simulink model "VCU_CS75_9_30"  (R2014a)
settings: Solver=FixedStepDiscrete  StartTime=0.0  StopTime=25  FixedStep=0.0005  RelTol=1e-3
undefined symbols (not defined in the file or in its folder): APAStatus_2D4, ecucoder_acal, I_SW01_L, LDW, ST_comd, TX2D4
libraries: simulink x881, ec5744lib x37
(part 4 of 30)

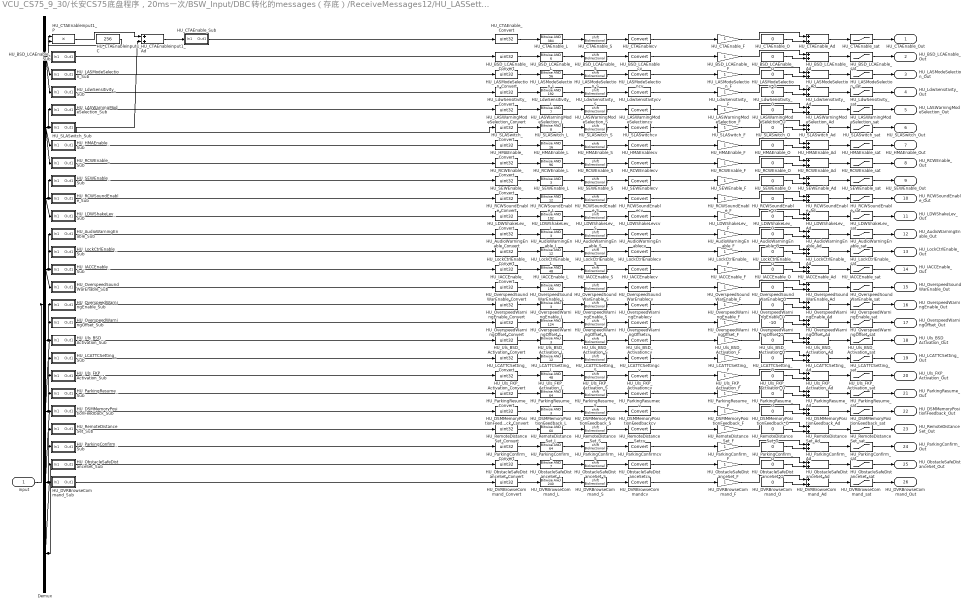
== system VCU_CS75_9_30/长安CS75底盘程序，20ms一次/BSW_Input/DBC转化的messages（存底）/ReceiveMessages12/HU_LASSetting_0x541 ==
  input : Inport
  Demux : Demux  Outputs=8
  HU_AudioWarningEnable_Ad : Sum
  HU_AudioWarningEnable_Convert : DataTypeConversion  OutDataTypeStr=uint32
  HU_AudioWarningEnable_F : Gain
  HU_AudioWarningEnable_L : simulink/Logic and Bit Operations/Bitwise Operator  logicop=AND  UseBitMask=on  BitMask=3  BitMaskRealWorld=Stored Integer
  HU_AudioWarningEnable_O : Constant  Value=0  OutDataTypeStr=single
  HU_AudioWarningEnable_S : ArithShift
  HU_AudioWarningEnable_Sub : Subsystem
  HU_AudioWarningEnable_sat : Saturate  UpperLimit=3  LowerLimit=0
  HU_AudioWarningEnablecv : DataTypeConversion
  HU_BSD_LCAEnable_Ad : Sum
  HU_BSD_LCAEnable_Convert : DataTypeConversion  OutDataTypeStr=uint32
  HU_BSD_LCAEnable_F : Gain
  HU_BSD_LCAEnable_L : simulink/Logic and Bit Operations/Bitwise Operator  logicop=AND  UseBitMask=on  BitMask=6  BitMaskRealWorld=Stored Integer
  HU_BSD_LCAEnable_O : Constant  Value=0  OutDataTypeStr=single
  HU_BSD_LCAEnable_S : ArithShift  BitShiftNumber=1
  HU_BSD_LCAEnable_Sub : Subsystem
  HU_BSD_LCAEnable_sat : Saturate  UpperLimit=3  LowerLimit=0
  HU_BSD_LCAEnablecv : DataTypeConversion
  HU_CTAEnable_Ad : Sum
  HU_CTAEnable_Convert : DataTypeConversion  OutDataTypeStr=uint32
  HU_CTAEnable_F : Gain
  HU_CTAEnable_L : simulink/Logic and Bit Operations/Bitwise Operator  logicop=AND  UseBitMask=on  BitMask=384  BitMaskRealWorld=Stored Integer
  HU_CTAEnable_O : Constant  Value=0  OutDataTypeStr=single
  HU_CTAEnable_S : ArithShift  BitShiftNumber=7
  HU_CTAEnable_Sub : Subsystem
  HU_CTAEnable_sat : Saturate  UpperLimit=3  LowerLimit=0
  HU_CTAEnablecv : DataTypeConversion
  HU_CTAEnableinput1_Ad : Sum
  HU_CTAEnableinput1_C : Constant  Value=256
  HU_CTAEnableinput1_P : Product
  HU_DSMMemoryPositionFeedback_Ad : Sum
  HU_DSMMemoryPositionFeedback_Convert : DataTypeConversion  OutDataTypeStr=uint32
  HU_DSMMemoryPositionFeedback_F : Gain
  HU_DSMMemoryPositionFeedback_L : simulink/Logic and Bit Operations/Bitwise Operator  logicop=AND  UseBitMask=on  BitMask=3  BitMaskRealWorld=Stored Integer
  HU_DSMMemoryPositionFeedback_O : Constant  Value=0  OutDataTypeStr=single
  HU_DSMMemoryPositionFeedback_S : ArithShift
  HU_DSMMemoryPositionFeedback_Sub : Subsystem
  HU_DSMMemoryPositionFeedback_sat : Saturate  UpperLimit=3  LowerLimit=0
  HU_DSMMemoryPositionFeedbackcv : DataTypeConversion
  HU_DVRBrowseCommand_Ad : Sum
  HU_DVRBrowseCommand_Convert : DataTypeConversion  OutDataTypeStr=uint32
  HU_DVRBrowseCommand_F : Gain
  HU_DVRBrowseCommand_L : simulink/Logic and Bit Operations/Bitwise Operator  logicop=AND  UseBitMask=on  BitMask=240  BitMaskRealWorld=Stored Integer
  HU_DVRBrowseCommand_O : Constant  Value=0  OutDataTypeStr=single
  HU_DVRBrowseCommand_S : ArithShift  BitShiftNumber=4
  HU_DVRBrowseCommand_Sub : Subsystem
  HU_DVRBrowseCommand_sat : Saturate  UpperLimit=15  LowerLimit=0
  HU_DVRBrowseCommandcv : DataTypeConversion
  HU_HMAEnable_Ad : Sum
  HU_HMAEnable_Convert : DataTypeConversion  OutDataTypeStr=uint32
  HU_HMAEnable_F : Gain
  HU_HMAEnable_L : simulink/Logic and Bit Operations/Bitwise Operator  logicop=AND  UseBitMask=on  BitMask=16  BitMaskRealWorld=Stored Integer
  HU_HMAEnable_O : Constant  Value=0  OutDataTypeStr=single
  HU_HMAEnable_S : ArithShift  BitShiftNumber=4
  HU_HMAEnable_Sub : Subsystem
  HU_HMAEnable_sat : Saturate  UpperLimit=1  LowerLimit=0
  HU_HMAEnablecv : DataTypeConversion
  HU_IACCEnable_Ad : Sum
  HU_IACCEnable_Convert : DataTypeConversion  OutDataTypeStr=uint32
  HU_IACCEnable_F : Gain
  HU_IACCEnable_L : simulink/Logic and Bit Operations/Bitwise Operator  logicop=AND  UseBitMask=on  BitMask=48  BitMaskRealWorld=Stored Integer
  HU_IACCEnable_O : Constant  Value=0  OutDataTypeStr=single
  HU_IACCEnable_S : ArithShift  BitShiftNumber=4
  HU_IACCEnable_Sub : Subsystem
  HU_IACCEnable_sat : Saturate  UpperLimit=3  LowerLimit=0
  HU_IACCEnablecv : DataTypeConversion
  HU_LASModeSelection_Ad : Sum
  HU_LASModeSelection_Convert : DataTypeConversion  OutDataTypeStr=uint32
  HU_LASModeSelection_F : Gain
  HU_LASModeSelection_L : simulink/Logic and Bit Operations/Bitwise Operator  logicop=AND  UseBitMask=on  BitMask=56  BitMaskRealWorld=Stored Integer
  HU_LASModeSelection_O : Constant  Value=0  OutDataTypeStr=single
  HU_LASModeSelection_S : ArithShift  BitShiftNumber=3
  HU_LASModeSelection_Sub : Subsystem
  HU_LASModeSelection_sat : Saturate  UpperLimit=7  LowerLimit=0
  HU_LASModeSelectioncv : DataTypeConversion
  HU_LASWarningModeSelection_Ad : Sum
  HU_LASWarningModeSelection_Convert : DataTypeConversion  OutDataTypeStr=uint32
  HU_LASWarningModeSelection_F : Gain
  HU_LASWarningModeSelection_L : simulink/Logic and Bit Operations/Bitwise Operator  logicop=AND  UseBitMask=on  BitMask=7  BitMaskRealWorld=Stored Integer
  HU_LASWarningModeSelection_O : Constant  Value=0  OutDataTypeStr=single
  HU_LASWarningModeSelection_S : ArithShift
  HU_LASWarningModeSelection_Sub : Subsystem
  HU_LASWarningModeSelection_sat : Saturate  UpperLimit=7  LowerLimit=0
  HU_LASWarningModeSelectioncv : DataTypeConversion
  HU_LCATTCSetting_Ad : Sum
  HU_LCATTCSetting_Convert : DataTypeConversion  OutDataTypeStr=uint32
  HU_LCATTCSetting_F : Gain
  HU_LCATTCSetting_L : simulink/Logic and Bit Operations/Bitwise Operator  logicop=AND  UseBitMask=on  BitMask=12  BitMaskRealWorld=Stored Integer
  HU_LCATTCSetting_O : Constant  Value=0  OutDataTypeStr=single
  HU_LCATTCSetting_S : ArithShift  BitShiftNumber=2
  HU_LCATTCSetting_Sub : Subsystem
  HU_LCATTCSetting_sat : Saturate  UpperLimit=3  LowerLimit=0
  HU_LCATTCSettingcv : DataTypeConversion
  HU_LDWShakeLev_Ad : Sum
  HU_LDWShakeLev_Convert : DataTypeConversion  OutDataTypeStr=uint32
  HU_LDWShakeLev_F : Gain
  HU_LDWShakeLev_L : simulink/Logic and Bit Operations/Bitwise Operator  logicop=AND  UseBitMask=on  BitMask=192  BitMaskRealWorld=Stored Integer
  HU_LDWShakeLev_O : Constant  Value=0  OutDataTypeStr=single
  HU_LDWShakeLev_S : ArithShift  BitShiftNumber=6
  HU_LDWShakeLev_Sub : Subsystem
  HU_LDWShakeLev_sat : Saturate  UpperLimit=3  LowerLimit=0
  HU_LDWShakeLevcv : DataTypeConversion
  HU_LdwSensitivity_Ad : Sum
  HU_LdwSensitivity_Convert : DataTypeConversion  OutDataTypeStr=uint32
  HU_LdwSensitivity_F : Gain
  HU_LdwSensitivity_L : simulink/Logic and Bit Operations/Bitwise Operator  logicop=AND  UseBitMask=on  BitMask=192  BitMaskRealWorld=Stored Integer
  HU_LdwSensitivity_O : Constant  Value=0  OutDataTypeStr=single
  HU_LdwSensitivity_S : ArithShift  BitShiftNumber=6
  HU_LdwSensitivity_Sub : Subsystem
  HU_LdwSensitivity_sat : Saturate  UpperLimit=3  LowerLimit=0
  HU_LdwSensitivitycv : DataTypeConversion
  HU_LockCtrlEnable_Ad : Sum
  HU_LockCtrlEnable_Convert : DataTypeConversion  OutDataTypeStr=uint32
  HU_LockCtrlEnable_F : Gain
  HU_LockCtrlEnable_L : simulink/Logic and Bit Operations/Bitwise Operator  logicop=AND  UseBitMask=on  BitMask=12  BitMaskRealWorld=Stored Integer
  HU_LockCtrlEnable_O : Constant  Value=0  OutDataTypeStr=single
  HU_LockCtrlEnable_S : ArithShift  BitShiftNumber=2
  HU_LockCtrlEnable_Sub : Subsystem
  HU_LockCtrlEnable_sat : Saturate  UpperLimit=3  LowerLimit=0
  HU_LockCtrlEnablecv : DataTypeConversion
  HU_ObstacleSafeDistanceSet_Ad : Sum
  HU_ObstacleSafeDistanceSet_Convert : DataTypeConversion  OutDataTypeStr=uint32
  HU_ObstacleSafeDistanceSet_F : Gain
  HU_ObstacleSafeDistanceSet_L : simulink/Logic and Bit Operations/Bitwise Operator  logicop=AND  UseBitMask=on  BitMask=7  BitMaskRealWorld=Stored Integer
  HU_ObstacleSafeDistanceSet_O : Constant  Value=0  OutDataTypeStr=single
  HU_ObstacleSafeDistanceSet_S : ArithShift
  HU_ObstacleSafeDistanceSet_Sub : Subsystem
  HU_ObstacleSafeDistanceSet_sat : Saturate  UpperLimit=7  LowerLimit=0
  HU_ObstacleSafeDistanceSetcv : DataTypeConversion
  HU_OverspeedSoundWarEnable_Ad : Sum
  HU_OverspeedSoundWarEnable_Convert : DataTypeConversion  OutDataTypeStr=uint32
  HU_OverspeedSoundWarEnable_F : Gain
  HU_OverspeedSoundWarEnable_L : simulink/Logic and Bit Operations/Bitwise Operator  logicop=AND  UseBitMask=on  BitMask=192  BitMaskRealWorld=Stored Integer
  HU_OverspeedSoundWarEnable_O : Constant  Value=0  OutDataTypeStr=single
  HU_OverspeedSoundWarEnable_S : ArithShift  BitShiftNumber=6
  HU_OverspeedSoundWarEnable_Sub : Subsystem
  HU_OverspeedSoundWarEnable_sat : Saturate  UpperLimit=3  LowerLimit=0
  HU_OverspeedSoundWarEnablecv : DataTypeConversion
  HU_OverspeedWarningEnable_Ad : Sum
  HU_OverspeedWarningEnable_Convert : DataTypeConversion  OutDataTypeStr=uint32
  HU_OverspeedWarningEnable_F : Gain
  HU_OverspeedWarningEnable_L : simulink/Logic and Bit Operations/Bitwise Operator  logicop=AND  UseBitMask=on  BitMask=3  BitMaskRealWorld=Stored Integer
  HU_OverspeedWarningEnable_O : Constant  Value=0  OutDataTypeStr=single
  HU_OverspeedWarningEnable_S : ArithShift
  HU_OverspeedWarningEnable_Sub : Subsystem
  HU_OverspeedWarningEnable_sat : Saturate  UpperLimit=3  LowerLimit=0
  HU_OverspeedWarningEnablecv : DataTypeConversion
  HU_OverspeedWarningOffset_Ad : Sum
  HU_OverspeedWarningOffset_Convert : DataTypeConversion  OutDataTypeStr=uint32
  HU_OverspeedWarningOffset_F : Gain
  HU_OverspeedWarningOffset_L : simulink/Logic and Bit Operations/Bitwise Operator  logicop=AND  UseBitMask=on  BitMask=124  BitMaskRealWorld=Stored Integer
  HU_OverspeedWarningOffset_O : Constant  Value=-10  OutDataTypeStr=single
  HU_OverspeedWarningOffset_S : ArithShift  BitShiftNumber=2
  HU_OverspeedWarningOffset_Sub : Subsystem
  HU_OverspeedWarningOffset_sat : Saturate  UpperLimit=10  LowerLimit=-10
  HU_OverspeedWarningOffsetcv : DataTypeConversion
  HU_ParkingConfirm_Ad : Sum
  HU_ParkingConfirm_Convert : DataTypeConversion  OutDataTypeStr=uint32
  HU_ParkingConfirm_F : Gain
  HU_ParkingConfirm_L : simulink/Logic and Bit Operations/Bitwise Operator  logicop=AND  UseBitMask=on  BitMask=64  BitMaskRealWorld=Stored Integer
  HU_ParkingConfirm_O : Constant  Value=0  OutDataTypeStr=single
  HU_ParkingConfirm_S : ArithShift  BitShiftNumber=6
  HU_ParkingConfirm_Sub : Subsystem
  HU_ParkingConfirm_sat : Saturate  UpperLimit=1  LowerLimit=0
  HU_ParkingConfirmcv : DataTypeConversion
  HU_ParkingResume_Ad : Sum
  HU_ParkingResume_Convert : DataTypeConversion  OutDataTypeStr=uint32
  HU_ParkingResume_F : Gain
  HU_ParkingResume_L : simulink/Logic and Bit Operations/Bitwise Operator  logicop=AND  UseBitMask=on  BitMask=64  BitMaskRealWorld=Stored Integer
  HU_ParkingResume_O : Constant  Value=0  OutDataTypeStr=single
  HU_ParkingResume_S : ArithShift  BitShiftNumber=6
  HU_ParkingResume_Sub : Subsystem
  HU_ParkingResume_sat : Saturate  UpperLimit=1  LowerLimit=0
  HU_ParkingResumecv : DataTypeConversion
  HU_RCWEnable_Ad : Sum
  HU_RCWEnable_Convert : DataTypeConversion  OutDataTypeStr=uint32
  HU_RCWEnable_F : Gain
  HU_RCWEnable_L : simulink/Logic and Bit Operations/Bitwise Operator  logicop=AND  UseBitMask=on  BitMask=96  BitMaskRealWorld=Stored Integer
  HU_RCWEnable_O : Constant  Value=0  OutDataTypeStr=single
  HU_RCWEnable_S : ArithShift  BitShiftNumber=5
  HU_RCWEnable_Sub : Subsystem
  HU_RCWEnable_sat : Saturate  UpperLimit=3  LowerLimit=0
  HU_RCWEnablecv : DataTypeConversion
  HU_RCWSoundEnable_Ad : Sum
  HU_RCWSoundEnable_Convert : DataTypeConversion  OutDataTypeStr=uint32
  HU_RCWSoundEnable_F : Gain
  HU_RCWSoundEnable_L : simulink/Logic and Bit Operations/Bitwise Operator  logicop=AND  UseBitMask=on  BitMask=12  BitMaskRealWorld=Stored Integer
  HU_RCWSoundEnable_O : Constant  Value=0  OutDataTypeStr=single
  HU_RCWSoundEnable_S : ArithShift  BitShiftNumber=2
  HU_RCWSoundEnable_Sub : Subsystem
  HU_RCWSoundEnable_sat : Saturate  UpperLimit=3  LowerLimit=0
  HU_RCWSoundEnablecv : DataTypeConversion
  HU_RemoteDistanceSet_Ad : Sum
  HU_RemoteDistanceSet_Convert : DataTypeConversion  OutDataTypeStr=uint32
  HU_RemoteDistanceSet_F : Gain
  HU_RemoteDistanceSet_L : simulink/Logic and Bit Operations/Bitwise Operator  logicop=AND  UseBitMask=on  BitMask=60  BitMaskRealWorld=Stored Integer
  HU_RemoteDistanceSet_O : Constant  Value=0  OutDataTypeStr=single
  HU_RemoteDistanceSet_S : ArithShift  BitShiftNumber=2
  HU_RemoteDistanceSet_Sub : Subsystem
  HU_RemoteDistanceSet_sat : Saturate  UpperLimit=15  LowerLimit=0
  HU_RemoteDistanceSetcv : DataTypeConversion
  HU_SEWEnable_Ad : Sum
  HU_SEWEnable_Convert : DataTypeConversion  OutDataTypeStr=uint32
  HU_SEWEnable_F : Gain
  HU_SEWEnable_L : simulink/Logic and Bit Operations/Bitwise Operator  logicop=AND  UseBitMask=on  BitMask=3  BitMaskRealWorld=Stored Integer
  HU_SEWEnable_O : Constant  Value=0  OutDataTypeStr=single
  HU_SEWEnable_S : ArithShift
  HU_SEWEnable_Sub : Subsystem
  HU_SEWEnable_sat : Saturate  UpperLimit=3  LowerLimit=0
  HU_SEWEnablecv : DataTypeConversion
  HU_SLASwitch_Ad : Sum
  HU_SLASwitch_Convert : DataTypeConversion  OutDataTypeStr=uint32
  HU_SLASwitch_F : Gain
  HU_SLASwitch_L : simulink/Logic and Bit Operations/Bitwise Operator  logicop=AND  UseBitMask=on  BitMask=8  BitMaskRealWorld=Stored Integer
  HU_SLASwitch_O : Constant  Value=0  OutDataTypeStr=single
  HU_SLASwitch_S : ArithShift  BitShiftNumber=3
  HU_SLASwitch_Sub : Subsystem
  HU_SLASwitch_sat : Saturate  UpperLimit=1  LowerLimit=0
  HU_SLASwitchcv : DataTypeConversion
  HU_Uls_BSD_Activation_Ad : Sum
  HU_Uls_BSD_Activation_Convert : DataTypeConversion  OutDataTypeStr=uint32
  HU_Uls_BSD_Activation_F : Gain
  HU_Uls_BSD_Activation_L : simulink/Logic and Bit Operations/Bitwise Operator  logicop=AND  UseBitMask=on  BitMask=3  BitMaskRealWorld=Stored Integer
  HU_Uls_BSD_Activation_O : Constant  Value=0  OutDataTypeStr=single
  HU_Uls_BSD_Activation_S : ArithShift
  HU_Uls_BSD_Activation_Sub : Subsystem
  HU_Uls_BSD_Activation_sat : Saturate  UpperLimit=3  LowerLimit=0
  HU_Uls_BSD_Activationcv : DataTypeConversion
  HU_Uls_FKP_Activation_Ad : Sum
  HU_Uls_FKP_Activation_Convert : DataTypeConversion  OutDataTypeStr=uint32
  HU_Uls_FKP_Activation_F : Gain
  HU_Uls_FKP_Activation_L : simulink/Logic and Bit Operations/Bitwise Operator  logicop=AND  UseBitMask=on  BitMask=48  BitMaskRealWorld=Stored Integer
  HU_Uls_FKP_Activation_O : Constant  Value=0  OutDataTypeStr=single
  HU_Uls_FKP_Activation_S : ArithShift  BitShiftNumber=4
  HU_Uls_FKP_Activation_Sub : Subsystem
  HU_Uls_FKP_Activation_sat : Saturate  UpperLimit=3  LowerLimit=0
  HU_Uls_FKP_Activationcv : DataTypeConversion
  HU_CTAEnable_Out : Outport
  HU_BSD_LCAEnable_Out : Outport  Port=2
  HU_LASModeSelection_Out : Outport  Port=3
  HU_LdwSensitivity_Out : Outport  Port=4
  HU_LASWarningModeSelection_Out : Outport  Port=5
  HU_SLASwitch_Out : Outport  Port=6
  HU_HMAEnable_Out : Outport  Port=7
  HU_RCWEnable_Out : Outport  Port=8
  HU_SEWEnable_Out : Outport  Port=9
  HU_RCWSoundEnable_Out : Outport  Port=10
  HU_LDWShakeLev_Out : Outport  Port=11
  HU_AudioWarningEnable_Out : Outport  Port=12
  HU_LockCtrlEnable_Out : Outport  Port=13
  HU_IACCEnable_Out : Outport  Port=14
  HU_OverspeedSoundWarEnable_Out : Outport  Port=15
  HU_OverspeedWarningEnable_Out : Outport  Port=16
  HU_OverspeedWarningOffset_Out : Outport  Port=17
  HU_Uls_BSD_Activation_Out : Outport  Port=18
  HU_LCATTCSetting_Out : Outport  Port=19
  HU_Uls_FKP_Activation_Out : Outport  Port=20
  HU_ParkingResume_Out : Outport  Port=21
  HU_DSMMemoryPositionFeedback_Out : Outport  Port=22
  HU_RemoteDistanceSet_Out : Outport  Port=23
  HU_ParkingConfirm_Out : Outport  Port=24
  HU_ObstacleSafeDistanceSet_Out : Outport  Port=25
  HU_DVRBrowseCommand_Out : Outport  Port=26
  wires:
  input/1 -> Demux/1
  HU_DVRBrowseCommandcv/1 -> HU_DVRBrowseCommand_F/1
  HU_DVRBrowseCommand_S/1 -> HU_DVRBrowseCommandcv/1
  HU_DVRBrowseCommand_L/1 -> HU_DVRBrowseCommand_S/1
  HU_DVRBrowseCommand_Convert/1 -> HU_DVRBrowseCommand_L/1
  HU_DVRBrowseCommand_Sub/1(Out1) -> HU_DVRBrowseCommand_Convert/1
  HU_DVRBrowseCommand_sat/1 -> HU_DVRBrowseCommand_Out/1
  HU_DVRBrowseCommand_Ad/1 -> HU_DVRBrowseCommand_sat/1
  HU_DVRBrowseCommand_O/1 -> HU_DVRBrowseCommand_Ad/2
  HU_DVRBrowseCommand_F/1 -> HU_DVRBrowseCommand_Ad/1
  HU_ObstacleSafeDistanceSetcv/1 -> HU_ObstacleSafeDistanceSet_F/1
  HU_ObstacleSafeDistanceSet_S/1 -> HU_ObstacleSafeDistanceSetcv/1
  HU_ObstacleSafeDistanceSet_L/1 -> HU_ObstacleSafeDistanceSet_S/1
  HU_ObstacleSafeDistanceSet_Convert/1 -> HU_ObstacleSafeDistanceSet_L/1
  HU_ObstacleSafeDistanceSet_Sub/1(Out1) -> HU_ObstacleSafeDistanceSet_Convert/1
  Demux/8 -> HU_DVRBrowseCommand_Sub/1(In1), HU_ObstacleSafeDistanceSet_Sub/1(In1)
  HU_ObstacleSafeDistanceSet_sat/1 -> HU_ObstacleSafeDistanceSet_Out/1
  HU_ObstacleSafeDistanceSet_Ad/1 -> HU_ObstacleSafeDistanceSet_sat/1
  HU_ObstacleSafeDistanceSet_O/1 -> HU_ObstacleSafeDistanceSet_Ad/2
  HU_ObstacleSafeDistanceSet_F/1 -> HU_ObstacleSafeDistanceSet_Ad/1
  HU_ParkingConfirmcv/1 -> HU_ParkingConfirm_F/1
  HU_ParkingConfirm_S/1 -> HU_ParkingConfirmcv/1
  HU_ParkingConfirm_L/1 -> HU_ParkingConfirm_S/1
  HU_ParkingConfirm_Convert/1 -> HU_ParkingConfirm_L/1
  HU_ParkingConfirm_Sub/1(Out1) -> HU_ParkingConfirm_Convert/1
  HU_ParkingConfirm_sat/1 -> HU_ParkingConfirm_Out/1
  HU_ParkingConfirm_Ad/1 -> HU_ParkingConfirm_sat/1
  HU_ParkingConfirm_O/1 -> HU_ParkingConfirm_Ad/2
  HU_ParkingConfirm_F/1 -> HU_ParkingConfirm_Ad/1
  HU_RemoteDistanceSetcv/1 -> HU_RemoteDistanceSet_F/1
  HU_RemoteDistanceSet_S/1 -> HU_RemoteDistanceSetcv/1
  HU_RemoteDistanceSet_L/1 -> HU_RemoteDistanceSet_S/1
  HU_RemoteDistanceSet_Convert/1 -> HU_RemoteDistanceSet_L/1
  HU_RemoteDistanceSet_Sub/1(Out1) -> HU_RemoteDistanceSet_Convert/1
  HU_RemoteDistanceSet_sat/1 -> HU_RemoteDistanceSet_Out/1
  HU_RemoteDistanceSet_Ad/1 -> HU_RemoteDistanceSet_sat/1
  HU_RemoteDistanceSet_O/1 -> HU_RemoteDistanceSet_Ad/2
  HU_RemoteDistanceSet_F/1 -> HU_RemoteDistanceSet_Ad/1
  HU_DSMMemoryPositionFeedbackcv/1 -> HU_DSMMemoryPositionFeedback_F/1
  HU_DSMMemoryPositionFeedback_S/1 -> HU_DSMMemoryPositionFeedbackcv/1
  HU_DSMMemoryPositionFeedback_L/1 -> HU_DSMMemoryPositionFeedback_S/1
  HU_DSMMemoryPositionFeedback_Convert/1 -> HU_DSMMemoryPositionFeedback_L/1
  HU_DSMMemoryPositionFeedback_Sub/1(Out1) -> HU_DSMMemoryPositionFeedback_Convert/1
  Demux/7 -> HU_ParkingConfirm_Sub/1(In1), HU_RemoteDistanceSet_Sub/1(In1), HU_DSMMemoryPositionFeedback_Sub/1(In1)
  HU_DSMMemoryPositionFeedback_sat/1 -> HU_DSMMemoryPositionFeedback_Out/1
  HU_DSMMemoryPositionFeedback_Ad/1 -> HU_DSMMemoryPositionFeedback_sat/1
  HU_DSMMemoryPositionFeedback_O/1 -> HU_DSMMemoryPositionFeedback_Ad/2
  HU_DSMMemoryPositionFeedback_F/1 -> HU_DSMMemoryPositionFeedback_Ad/1
  HU_ParkingResumecv/1 -> HU_ParkingResume_F/1
  HU_ParkingResume_S/1 -> HU_ParkingResumecv/1
  HU_ParkingResume_L/1 -> HU_ParkingResume_S/1
  HU_ParkingResume_Convert/1 -> HU_ParkingResume_L/1
  HU_ParkingResume_Sub/1(Out1) -> HU_ParkingResume_Convert/1
  HU_ParkingResume_sat/1 -> HU_ParkingResume_Out/1
  HU_ParkingResume_Ad/1 -> HU_ParkingResume_sat/1
  HU_ParkingResume_O/1 -> HU_ParkingResume_Ad/2
  HU_ParkingResume_F/1 -> HU_ParkingResume_Ad/1
  HU_Uls_FKP_Activationcv/1 -> HU_Uls_FKP_Activation_F/1
  HU_Uls_FKP_Activation_S/1 -> HU_Uls_FKP_Activationcv/1
  HU_Uls_FKP_Activation_L/1 -> HU_Uls_FKP_Activation_S/1
  HU_Uls_FKP_Activation_Convert/1 -> HU_Uls_FKP_Activation_L/1
  HU_Uls_FKP_Activation_Sub/1(Out1) -> HU_Uls_FKP_Activation_Convert/1
  HU_Uls_FKP_Activation_sat/1 -> HU_Uls_FKP_Activation_Out/1
  HU_Uls_FKP_Activation_Ad/1 -> HU_Uls_FKP_Activation_sat/1
  HU_Uls_FKP_Activation_O/1 -> HU_Uls_FKP_Activation_Ad/2
  HU_Uls_FKP_Activation_F/1 -> HU_Uls_FKP_Activation_Ad/1
  HU_LCATTCSettingcv/1 -> HU_LCATTCSetting_F/1
  HU_LCATTCSetting_S/1 -> HU_LCATTCSettingcv/1
  HU_LCATTCSetting_L/1 -> HU_LCATTCSetting_S/1
  HU_LCATTCSetting_Convert/1 -> HU_LCATTCSetting_L/1
  HU_LCATTCSetting_Sub/1(Out1) -> HU_LCATTCSetting_Convert/1
  HU_LCATTCSetting_sat/1 -> HU_LCATTCSetting_Out/1
  HU_LCATTCSetting_Ad/1 -> HU_LCATTCSetting_sat/1
  HU_LCATTCSetting_O/1 -> HU_LCATTCSetting_Ad/2
  HU_LCATTCSetting_F/1 -> HU_LCATTCSetting_Ad/1
  HU_Uls_BSD_Activationcv/1 -> HU_Uls_BSD_Activation_F/1
  HU_Uls_BSD_Activation_S/1 -> HU_Uls_BSD_Activationcv/1
  HU_Uls_BSD_Activation_L/1 -> HU_Uls_BSD_Activation_S/1
  HU_Uls_BSD_Activation_Convert/1 -> HU_Uls_BSD_Activation_L/1
  HU_Uls_BSD_Activation_Sub/1(Out1) -> HU_Uls_BSD_Activation_Convert/1
  Demux/6 -> HU_ParkingResume_Sub/1(In1), HU_Uls_FKP_Activation_Sub/1(In1), HU_LCATTCSetting_Sub/1(In1), HU_Uls_BSD_Activation_Sub/1(In1)
  HU_Uls_BSD_Activation_sat/1 -> HU_Uls_BSD_Activation_Out/1
  HU_Uls_BSD_Activation_Ad/1 -> HU_Uls_BSD_Activation_sat/1
  HU_Uls_BSD_Activation_O/1 -> HU_Uls_BSD_Activation_Ad/2
  HU_Uls_BSD_Activation_F/1 -> HU_Uls_BSD_Activation_Ad/1
  HU_OverspeedWarningOffsetcv/1 -> HU_OverspeedWarningOffset_F/1
  HU_OverspeedWarningOffset_S/1 -> HU_OverspeedWarningOffsetcv/1
  HU_OverspeedWarningOffset_L/1 -> HU_OverspeedWarningOffset_S/1
  HU_OverspeedWarningOffset_Convert/1 -> HU_OverspeedWarningOffset_L/1
  HU_OverspeedWarningOffset_Sub/1(Out1) -> HU_OverspeedWarningOffset_Convert/1
  HU_OverspeedWarningOffset_sat/1 -> HU_OverspeedWarningOffset_Out/1
  HU_OverspeedWarningOffset_Ad/1 -> HU_OverspeedWarningOffset_sat/1
  HU_OverspeedWarningOffset_O/1 -> HU_OverspeedWarningOffset_Ad/2
  HU_OverspeedWarningOffset_F/1 -> HU_OverspeedWarningOffset_Ad/1
  HU_OverspeedWarningEnablecv/1 -> HU_OverspeedWarningEnable_F/1
  HU_OverspeedWarningEnable_S/1 -> HU_OverspeedWarningEnablecv/1
  HU_OverspeedWarningEnable_L/1 -> HU_OverspeedWarningEnable_S/1
  HU_OverspeedWarningEnable_Convert/1 -> HU_OverspeedWarningEnable_L/1
  HU_OverspeedWarningEnable_Sub/1(Out1) -> HU_OverspeedWarningEnable_Convert/1
  Demux/5 -> HU_OverspeedWarningOffset_Sub/1(In1), HU_OverspeedWarningEnable_Sub/1(In1)
  HU_OverspeedWarningEnable_sat/1 -> HU_OverspeedWarningEnable_Out/1
  HU_OverspeedWarningEnable_Ad/1 -> HU_OverspeedWarningEnable_sat/1
  HU_OverspeedWarningEnable_O/1 -> HU_OverspeedWarningEnable_Ad/2
  HU_OverspeedWarningEnable_F/1 -> HU_OverspeedWarningEnable_Ad/1
  HU_OverspeedSoundWarEnablecv/1 -> HU_OverspeedSoundWarEnable_F/1
  HU_OverspeedSoundWarEnable_S/1 -> HU_OverspeedSoundWarEnablecv/1
  HU_OverspeedSoundWarEnable_L/1 -> HU_OverspeedSoundWarEnable_S/1
  HU_OverspeedSoundWarEnable_Convert/1 -> HU_OverspeedSoundWarEnable_L/1
  HU_OverspeedSoundWarEnable_Sub/1(Out1) -> HU_OverspeedSoundWarEnable_Convert/1
  HU_OverspeedSoundWarEnable_sat/1 -> HU_OverspeedSoundWarEnable_Out/1
  HU_OverspeedSoundWarEnable_Ad/1 -> HU_OverspeedSoundWarEnable_sat/1
  HU_OverspeedSoundWarEnable_O/1 -> HU_OverspeedSoundWarEnable_Ad/2
  HU_OverspeedSoundWarEnable_F/1 -> HU_OverspeedSoundWarEnable_Ad/1
  HU_IACCEnablecv/1 -> HU_IACCEnable_F/1
  HU_IACCEnable_S/1 -> HU_IACCEnablecv/1
  HU_IACCEnable_L/1 -> HU_IACCEnable_S/1
  HU_IACCEnable_Convert/1 -> HU_IACCEnable_L/1
  HU_IACCEnable_Sub/1(Out1) -> HU_IACCEnable_Convert/1
  HU_IACCEnable_sat/1 -> HU_IACCEnable_Out/1
  HU_IACCEnable_Ad/1 -> HU_IACCEnable_sat/1
  HU_IACCEnable_O/1 -> HU_IACCEnable_Ad/2
  HU_IACCEnable_F/1 -> HU_IACCEnable_Ad/1
  HU_LockCtrlEnablecv/1 -> HU_LockCtrlEnable_F/1
  HU_LockCtrlEnable_S/1 -> HU_LockCtrlEnablecv/1
  HU_LockCtrlEnable_L/1 -> HU_LockCtrlEnable_S/1
  HU_LockCtrlEnable_Convert/1 -> HU_LockCtrlEnable_L/1
  HU_LockCtrlEnable_Sub/1(Out1) -> HU_LockCtrlEnable_Convert/1
  HU_LockCtrlEnable_sat/1 -> HU_LockCtrlEnable_Out/1
  HU_LockCtrlEnable_Ad/1 -> HU_LockCtrlEnable_sat/1
  HU_LockCtrlEnable_O/1 -> HU_LockCtrlEnable_Ad/2
  HU_LockCtrlEnable_F/1 -> HU_LockCtrlEnable_Ad/1
  HU_AudioWarningEnablecv/1 -> HU_AudioWarningEnable_F/1
  HU_AudioWarningEnable_S/1 -> HU_AudioWarningEnablecv/1
  HU_AudioWarningEnable_L/1 -> HU_AudioWarningEnable_S/1
  HU_AudioWarningEnable_Convert/1 -> HU_AudioWarningEnable_L/1
  HU_AudioWarningEnable_Sub/1(Out1) -> HU_AudioWarningEnable_Convert/1
  Demux/4 -> HU_OverspeedSoundWarEnable_Sub/1(In1), HU_IACCEnable_Sub/1(In1), HU_LockCtrlEnable_Sub/1(In1), HU_AudioWarningEnable_Sub/1(In1)
  HU_AudioWarningEnable_sat/1 -> HU_AudioWarningEnable_Out/1
  HU_AudioWarningEnable_Ad/1 -> HU_AudioWarningEnable_sat/1
  HU_AudioWarningEnable_O/1 -> HU_AudioWarningEnable_Ad/2
  HU_AudioWarningEnable_F/1 -> HU_AudioWarningEnable_Ad/1
  HU_LDWShakeLevcv/1 -> HU_LDWShakeLev_F/1
  HU_LDWShakeLev_S/1 -> HU_LDWShakeLevcv/1
  HU_LDWShakeLev_L/1 -> HU_LDWShakeLev_S/1
  HU_LDWShakeLev_Convert/1 -> HU_LDWShakeLev_L/1
  HU_LDWShakeLev_Sub/1(Out1) -> HU_LDWShakeLev_Convert/1
  HU_LDWShakeLev_sat/1 -> HU_LDWShakeLev_Out/1
  HU_LDWShakeLev_Ad/1 -> HU_LDWShakeLev_sat/1
  HU_LDWShakeLev_O/1 -> HU_LDWShakeLev_Ad/2
  HU_LDWShakeLev_F/1 -> HU_LDWShakeLev_Ad/1
  HU_RCWSoundEnablecv/1 -> HU_RCWSoundEnable_F/1
  HU_RCWSoundEnable_S/1 -> HU_RCWSoundEnablecv/1
  HU_RCWSoundEnable_L/1 -> HU_RCWSoundEnable_S/1
  HU_RCWSoundEnable_Convert/1 -> HU_RCWSoundEnable_L/1
  HU_RCWSoundEnable_Sub/1(Out1) -> HU_RCWSoundEnable_Convert/1
  HU_RCWSoundEnable_sat/1 -> HU_RCWSoundEnable_Out/1
  HU_RCWSoundEnable_Ad/1 -> HU_RCWSoundEnable_sat/1
  HU_RCWSoundEnable_O/1 -> HU_RCWSoundEnable_Ad/2
  HU_RCWSoundEnable_F/1 -> HU_RCWSoundEnable_Ad/1
  HU_SEWEnablecv/1 -> HU_SEWEnable_F/1
  HU_SEWEnable_S/1 -> HU_SEWEnablecv/1
  HU_SEWEnable_L/1 -> HU_SEWEnable_S/1
  HU_SEWEnable_Convert/1 -> HU_SEWEnable_L/1
  HU_SEWEnable_Sub/1(Out1) -> HU_SEWEnable_Convert/1
  Demux/3 -> HU_LDWShakeLev_Sub/1(In1), HU_RCWSoundEnable_Sub/1(In1), HU_SEWEnable_Sub/1(In1)
  HU_SEWEnable_sat/1 -> HU_SEWEnable_Out/1
  HU_SEWEnable_Ad/1 -> HU_SEWEnable_sat/1
  HU_SEWEnable_O/1 -> HU_SEWEnable_Ad/2
  HU_SEWEnable_F/1 -> HU_SEWEnable_Ad/1
  HU_RCWEnablecv/1 -> HU_RCWEnable_F/1
  HU_RCWEnable_S/1 -> HU_RCWEnablecv/1
  HU_RCWEnable_L/1 -> HU_RCWEnable_S/1
  HU_RCWEnable_Convert/1 -> HU_RCWEnable_L/1
  HU_RCWEnable_Sub/1(Out1) -> HU_RCWEnable_Convert/1
  HU_RCWEnable_sat/1 -> HU_RCWEnable_Out/1
  HU_RCWEnable_Ad/1 -> HU_RCWEnable_sat/1
  HU_RCWEnable_O/1 -> HU_RCWEnable_Ad/2
  HU_RCWEnable_F/1 -> HU_RCWEnable_Ad/1
  HU_HMAEnablecv/1 -> HU_HMAEnable_F/1
  HU_HMAEnable_S/1 -> HU_HMAEnablecv/1
  HU_HMAEnable_L/1 -> HU_HMAEnable_S/1
  HU_HMAEnable_Convert/1 -> HU_HMAEnable_L/1
  HU_HMAEnable_Sub/1(Out1) -> HU_HMAEnable_Convert/1
  HU_HMAEnable_sat/1 -> HU_HMAEnable_Out/1
  HU_HMAEnable_Ad/1 -> HU_HMAEnable_sat/1
  HU_HMAEnable_O/1 -> HU_HMAEnable_Ad/2
  HU_HMAEnable_F/1 -> HU_HMAEnable_Ad/1
  HU_SLASwitchcv/1 -> HU_SLASwitch_F/1
  HU_SLASwitch_S/1 -> HU_SLASwitchcv/1
  HU_SLASwitch_L/1 -> HU_SLASwitch_S/1
  HU_SLASwitch_Convert/1 -> HU_SLASwitch_L/1
  HU_SLASwitch_Sub/1(Out1) -> HU_SLASwitch_Convert/1
  HU_SLASwitch_sat/1 -> HU_SLASwitch_Out/1
  HU_SLASwitch_Ad/1 -> HU_SLASwitch_sat/1
  HU_SLASwitch_O/1 -> HU_SLASwitch_Ad/2
  HU_SLASwitch_F/1 -> HU_SLASwitch_Ad/1
  HU_LASWarningModeSelectioncv/1 -> HU_LASWarningModeSelection_F/1
  HU_LASWarningModeSelection_S/1 -> HU_LASWarningModeSelectioncv/1
  HU_LASWarningModeSelection_L/1 -> HU_LASWarningModeSelection_S/1
  HU_LASWarningModeSelection_Convert/1 -> HU_LASWarningModeSelection_L/1
  HU_LASWarningModeSelection_Sub/1(Out1) -> HU_LASWarningModeSelection_Convert/1
  HU_LASWarningModeSelection_sat/1 -> HU_LASWarningModeSelection_Out/1
  HU_LASWarningModeSelection_Ad/1 -> HU_LASWarningModeSelection_sat/1
  HU_LASWarningModeSelection_O/1 -> HU_LASWarningModeSelection_Ad/2
  HU_LASWarningModeSelection_F/1 -> HU_LASWarningModeSelection_Ad/1
  HU_LdwSensitivitycv/1 -> HU_LdwSensitivity_F/1
  HU_LdwSensitivity_S/1 -> HU_LdwSensitivitycv/1
  HU_LdwSensitivity_L/1 -> HU_LdwSensitivity_S/1
  HU_LdwSensitivity_Convert/1 -> HU_LdwSensitivity_L/1
  HU_LdwSensitivity_Sub/1(Out1) -> HU_LdwSensitivity_Convert/1
  HU_LdwSensitivity_sat/1 -> HU_LdwSensitivity_Out/1
  HU_LdwSensitivity_Ad/1 -> HU_LdwSensitivity_sat/1
  HU_LdwSensitivity_O/1 -> HU_LdwSensitivity_Ad/2
  HU_LdwSensitivity_F/1 -> HU_LdwSensitivity_Ad/1
  HU_LASModeSelectioncv/1 -> HU_LASModeSelection_F/1
  HU_LASModeSelection_S/1 -> HU_LASModeSelectioncv/1
  HU_LASModeSelection_L/1 -> HU_LASModeSelection_S/1
  HU_LASModeSelection_Convert/1 -> HU_LASModeSelection_L/1
  HU_LASModeSelection_Sub/1(Out1) -> HU_LASModeSelection_Convert/1
  HU_LASModeSelection_sat/1 -> HU_LASModeSelection_Out/1
  HU_LASModeSelection_Ad/1 -> HU_LASModeSelection_sat/1
  HU_LASModeSelection_O/1 -> HU_LASModeSelection_Ad/2
  HU_LASModeSelection_F/1 -> HU_LASModeSelection_Ad/1
  HU_BSD_LCAEnablecv/1 -> HU_BSD_LCAEnable_F/1
  HU_BSD_LCAEnable_S/1 -> HU_BSD_LCAEnablecv/1
  HU_BSD_LCAEnable_L/1 -> HU_BSD_LCAEnable_S/1
  HU_BSD_LCAEnable_Convert/1 -> HU_BSD_LCAEnable_L/1
  HU_BSD_LCAEnable_Sub/1(Out1) -> HU_BSD_LCAEnable_Convert/1
  HU_BSD_LCAEnable_sat/1 -> HU_BSD_LCAEnable_Out/1
  HU_BSD_LCAEnable_Ad/1 -> HU_BSD_LCAEnable_sat/1
  HU_BSD_LCAEnable_O/1 -> HU_BSD_LCAEnable_Ad/2
  HU_BSD_LCAEnable_F/1 -> HU_BSD_LCAEnable_Ad/1
  HU_CTAEnablecv/1 -> HU_CTAEnable_F/1
  HU_CTAEnable_S/1 -> HU_CTAEnablecv/1
  HU_CTAEnable_L/1 -> HU_CTAEnable_S/1
  HU_CTAEnable_Convert/1 -> HU_CTAEnable_L/1
  HU_CTAEnable_Sub/1(Out1) -> HU_CTAEnable_Convert/1
  HU_CTAEnableinput1_Ad/1 -> HU_CTAEnable_Sub/1(In1)
  Demux/2 -> HU_RCWEnable_Sub/1(In1), HU_HMAEnable_Sub/1(In1), HU_SLASwitch_Sub/1(In1), HU_LASWarningModeSelection_Sub/1(In1), HU_CTAEnableinput1_Ad/2
  HU_CTAEnableinput1_P/1 -> HU_CTAEnableinput1_Ad/1
  HU_CTAEnableinput1_C/1 -> HU_CTAEnableinput1_P/2
  Demux/1 -> HU_LdwSensitivity_Sub/1(In1), HU_LASModeSelection_Sub/1(In1), HU_BSD_LCAEnable_Sub/1(In1), HU_CTAEnableinput1_P/1
  HU_CTAEnable_sat/1 -> HU_CTAEnable_Out/1
  HU_CTAEnable_Ad/1 -> HU_CTAEnable_sat/1
  HU_CTAEnable_O/1 -> HU_CTAEnable_Ad/2
  HU_CTAEnable_F/1 -> HU_CTAEnable_Ad/1

== system VCU_CS75_9_30/长安CS75底盘程序，20ms一次/BSW_Input/DBC转化的messages（存底）/ReceiveMessages13/SAS_108 ==
  input : Inport
  Demux : Demux  Outputs=8
  SAS_CRCCheck_Ad : Sum
  SAS_CRCCheck_Convert : DataTypeConversion  OutDataTypeStr=uint32
  SAS_CRCCheck_F : Gain
  SAS_CRCCheck_L : simulink/Logic and Bit Operations/Bitwise Operator  logicop=AND  UseBitMask=on  BitMask=255  BitMaskRealWorld=Stored Integer
  SAS_CRCCheck_O : Constant  Value=0  OutDataTypeStr=single
  SAS_CRCCheck_S : ArithShift
  SAS_CRCCheck_Sub : Subsystem
  SAS_CRCCheck_sat : Saturate  UpperLimit=255  LowerLimit=0
  SAS_CRCCheckcv : DataTypeConversion
  SAS_Calibrated_Ad : Sum
  SAS_Calibrated_Convert : DataTypeConversion  OutDataTypeStr=uint32
  SAS_Calibrated_F : Gain
  SAS_Calibrated_L : simulink/Logic and Bit Operations/Bitwise Operator  logicop=AND  UseBitMask=on  BitMask=32  BitMaskRealWorld=Stored Integer
  SAS_Calibrated_O : Constant  Value=0  OutDataTypeStr=single
  SAS_Calibrated_S : ArithShift  BitShiftNumber=5
  SAS_Calibrated_Sub : Subsystem
  SAS_Calibrated_sat : Saturate  UpperLimit=1  LowerLimit=0
  SAS_Calibratedcv : DataTypeConversion
  SAS_RollingCounter_Ad : Sum
  SAS_RollingCounter_Convert : DataTypeConversion  OutDataTypeStr=uint32
  SAS_RollingCounter_F : Gain
  SAS_RollingCounter_L : simulink/Logic and Bit Operations/Bitwise Operator  logicop=AND  UseBitMask=on  BitMask=15  BitMaskRealWorld=Stored Integer
  SAS_RollingCounter_O : Constant  Value=0  OutDataTypeStr=single
  SAS_RollingCounter_S : ArithShift
  SAS_RollingCounter_Sub : Subsystem
  SAS_RollingCounter_sat : Saturate  UpperLimit=15  LowerLimit=0
  SAS_RollingCountercv : DataTypeConversion
  SAS_SASFailure_Ad : Sum
  SAS_SASFailure_Convert : DataTypeConversion  OutDataTypeStr=uint32
  SAS_SASFailure_F : Gain
  SAS_SASFailure_L : simulink/Logic and Bit Operations/Bitwise Operator  logicop=AND  UseBitMask=on  BitMask=64  BitMaskRealWorld=Stored Integer
  SAS_SASFailure_O : Constant  Value=0  OutDataTypeStr=single
  SAS_SASFailure_S : ArithShift  BitShiftNumber=6
  SAS_SASFailure_Sub : Subsystem
  SAS_SASFailure_sat : Saturate  UpperLimit=1  LowerLimit=0
  SAS_SASFailurecv : DataTypeConversion
  SAS_SteeringAngleCS : ArithShift  BitShiftNumber=-16
  SAS_SteeringAngleCS1 : ArithShift  BitShiftNumber=-15
  SAS_SteeringAngleConS : Constant  OutDataTypeStr=single
  SAS_SteeringAngleMinus : UnaryMinus
  SAS_SteeringAngleROP : RelationalOperator  OutDataTypeStr=boolean
  SAS_SteeringAngleSW : Switch  Criteria=u2 ~= 0
  SAS_SteeringAngleSpeed_Ad : Sum
  SAS_SteeringAngleSpeed_Convert : DataTypeConversion  OutDataTypeStr=uint32
  SAS_SteeringAngleSpeed_F : Gain  Gain=4
  SAS_SteeringAngleSpeed_L : simulink/Logic and Bit Operations/Bitwise Operator  logicop=AND  UseBitMask=on  BitMask=255  BitMaskRealWorld=Stored Integer
  SAS_SteeringAngleSpeed_O : Constant  Value=0  OutDataTypeStr=single
  SAS_SteeringAngleSpeed_S : ArithShift
  SAS_SteeringAngleSpeed_Sub : Subsystem
  SAS_SteeringAngleSpeed_sat : Saturate  UpperLimit=1020  LowerLimit=0
  SAS_SteeringAngleSpeedcv : DataTypeConversion
  SAS_SteeringAngleValid_Ad : Sum
  SAS_SteeringAngleValid_Convert : DataTypeConversion  OutDataTypeStr=uint32
  SAS_SteeringAngleValid_F : Gain
  SAS_SteeringAngleValid_L : simulink/Logic and Bit Operations/Bitwise Operator  logicop=AND  UseBitMask=on  BitMask=128  BitMaskRealWorld=Stored Integer
  SAS_SteeringAngleValid_O : Constant  Value=0  OutDataTypeStr=single
  SAS_SteeringAngleValid_S : ArithShift  BitShiftNumber=7
  SAS_SteeringAngleValid_Sub : Subsystem
  SAS_SteeringAngleValid_sat : Saturate  UpperLimit=1  LowerLimit=0
  SAS_SteeringAngleValidcv : DataTypeConversion
  SAS_SteeringAngle_Ad : Sum
  SAS_SteeringAngle_Convert : DataTypeConversion  OutDataTypeStr=uint32
  SAS_SteeringAngle_F : Gain  Gain=0.1
  SAS_SteeringAngle_L : simulink/Logic and Bit Operations/Bitwise Operator  logicop=AND  UseBitMask=on  BitMask=65535  BitMaskRealWorld=Stored Integer
  SAS_SteeringAngle_O : Constant  Value=0  OutDataTypeStr=single
  SAS_SteeringAngle_S : ArithShift
  SAS_SteeringAngle_Sub : Subsystem
  SAS_SteeringAngle_sat : Saturate  UpperLimit=780  LowerLimit=-780
  SAS_SteeringAnglecv : DataTypeConversion
  SAS_SteeringAngleinput1_Ad : Sum
  SAS_SteeringAngleinput1_C : Constant  Value=256
  SAS_SteeringAngleinput1_P : Product
  SAS_SteeringAnglesubcon : Sum  Inputs=+-
  SAS_SteeringAngle_Out : Outport
  SAS_SteeringAngleSpeed_Out : Outport  Port=2
  SAS_Calibrated_Out : Outport  Port=3
  SAS_SASFailure_Out : Outport  Port=4
  SAS_SteeringAngleValid_Out : Outport  Port=5
  SAS_RollingCounter_Out : Outport  Port=6
  SAS_CRCCheck_Out : Outport  Port=7
  wires:
  input/1 -> Demux/1
  SAS_CRCCheckcv/1 -> SAS_CRCCheck_F/1
  SAS_CRCCheck_S/1 -> SAS_CRCCheckcv/1
  SAS_CRCCheck_L/1 -> SAS_CRCCheck_S/1
  SAS_CRCCheck_Convert/1 -> SAS_CRCCheck_L/1
  SAS_CRCCheck_Sub/1(Out1) -> SAS_CRCCheck_Convert/1
  Demux/8 -> SAS_CRCCheck_Sub/1(In1)
  SAS_CRCCheck_sat/1 -> SAS_CRCCheck_Out/1
  SAS_CRCCheck_Ad/1 -> SAS_CRCCheck_sat/1
  SAS_CRCCheck_O/1 -> SAS_CRCCheck_Ad/2
  SAS_CRCCheck_F/1 -> SAS_CRCCheck_Ad/1
  SAS_RollingCountercv/1 -> SAS_RollingCounter_F/1
  SAS_RollingCounter_S/1 -> SAS_RollingCountercv/1
  SAS_RollingCounter_L/1 -> SAS_RollingCounter_S/1
  SAS_RollingCounter_Convert/1 -> SAS_RollingCounter_L/1
  SAS_RollingCounter_Sub/1(Out1) -> SAS_RollingCounter_Convert/1
  Demux/7 -> SAS_RollingCounter_Sub/1(In1)
  SAS_RollingCounter_sat/1 -> SAS_RollingCounter_Out/1
  SAS_RollingCounter_Ad/1 -> SAS_RollingCounter_sat/1
  SAS_RollingCounter_O/1 -> SAS_RollingCounter_Ad/2
  SAS_RollingCounter_F/1 -> SAS_RollingCounter_Ad/1
  SAS_SteeringAngleValidcv/1 -> SAS_SteeringAngleValid_F/1
  SAS_SteeringAngleValid_S/1 -> SAS_SteeringAngleValidcv/1
  SAS_SteeringAngleValid_L/1 -> SAS_SteeringAngleValid_S/1
  SAS_SteeringAngleValid_Convert/1 -> SAS_SteeringAngleValid_L/1
  SAS_SteeringAngleValid_Sub/1(Out1) -> SAS_SteeringAngleValid_Convert/1
  SAS_SteeringAngleValid_sat/1 -> SAS_SteeringAngleValid_Out/1
  SAS_SteeringAngleValid_Ad/1 -> SAS_SteeringAngleValid_sat/1
  SAS_SteeringAngleValid_O/1 -> SAS_SteeringAngleValid_Ad/2
  SAS_SteeringAngleValid_F/1 -> SAS_SteeringAngleValid_Ad/1
  SAS_SASFailurecv/1 -> SAS_SASFailure_F/1
  SAS_SASFailure_S/1 -> SAS_SASFailurecv/1
  SAS_SASFailure_L/1 -> SAS_SASFailure_S/1
  SAS_SASFailure_Convert/1 -> SAS_SASFailure_L/1
  SAS_SASFailure_Sub/1(Out1) -> SAS_SASFailure_Convert/1
  SAS_SASFailure_sat/1 -> SAS_SASFailure_Out/1
  SAS_SASFailure_Ad/1 -> SAS_SASFailure_sat/1
  SAS_SASFailure_O/1 -> SAS_SASFailure_Ad/2
  SAS_SASFailure_F/1 -> SAS_SASFailure_Ad/1
  SAS_Calibratedcv/1 -> SAS_Calibrated_F/1
  SAS_Calibrated_S/1 -> SAS_Calibratedcv/1
  SAS_Calibrated_L/1 -> SAS_Calibrated_S/1
  SAS_Calibrated_Convert/1 -> SAS_Calibrated_L/1
  SAS_Calibrated_Sub/1(Out1) -> SAS_Calibrated_Convert/1
  Demux/4 -> SAS_SteeringAngleValid_Sub/1(In1), SAS_SASFailure_Sub/1(In1), SAS_Calibrated_Sub/1(In1)
  SAS_Calibrated_sat/1 -> SAS_Calibrated_Out/1
  SAS_Calibrated_Ad/1 -> SAS_Calibrated_sat/1
  SAS_Calibrated_O/1 -> SAS_Calibrated_Ad/2
  SAS_Calibrated_F/1 -> SAS_Calibrated_Ad/1
  SAS_SteeringAngleSpeedcv/1 -> SAS_SteeringAngleSpeed_F/1
  SAS_SteeringAngleSpeed_S/1 -> SAS_SteeringAngleSpeedcv/1
  SAS_SteeringAngleSpeed_L/1 -> SAS_SteeringAngleSpeed_S/1
  SAS_SteeringAngleSpeed_Convert/1 -> SAS_SteeringAngleSpeed_L/1
  SAS_SteeringAngleSpeed_Sub/1(Out1) -> SAS_SteeringAngleSpeed_Convert/1
  Demux/3 -> SAS_SteeringAngleSpeed_Sub/1(In1)
  SAS_SteeringAngleSpeed_sat/1 -> SAS_SteeringAngleSpeed_Out/1
  SAS_SteeringAngleSpeed_Ad/1 -> SAS_SteeringAngleSpeed_sat/1
  SAS_SteeringAngleSpeed_O/1 -> SAS_SteeringAngleSpeed_Ad/2
  SAS_SteeringAngleSpeed_F/1 -> SAS_SteeringAngleSpeed_Ad/1
  SAS_SteeringAngleROP/1 -> SAS_SteeringAngleSW/2
  SAS_SteeringAngleSW/1 -> SAS_SteeringAngle_F/1
  SAS_SteeringAngleMinus/1 -> SAS_SteeringAngleSW/1
  SAS_SteeringAnglesubcon/1 -> SAS_SteeringAngleMinus/1
  SAS_SteeringAngleCS/1 -> SAS_SteeringAnglesubcon/1
  SAS_SteeringAngleCS1/1 -> SAS_SteeringAngleROP/2
  SAS_SteeringAngleConS/1 -> SAS_SteeringAngleCS1/1, SAS_SteeringAngleCS/1
  SAS_SteeringAnglecv/1 -> SAS_SteeringAngleSW/3, SAS_SteeringAnglesubcon/2, SAS_SteeringAngleROP/1
  SAS_SteeringAngle_S/1 -> SAS_SteeringAnglecv/1
  SAS_SteeringAngle_L/1 -> SAS_SteeringAngle_S/1
  SAS_SteeringAngle_Convert/1 -> SAS_SteeringAngle_L/1
  SAS_SteeringAngle_Sub/1(Out1) -> SAS_SteeringAngle_Convert/1
  SAS_SteeringAngleinput1_Ad/1 -> SAS_SteeringAngle_Sub/1(In1)
  Demux/2 -> SAS_SteeringAngleinput1_Ad/2
  SAS_SteeringAngleinput1_P/1 -> SAS_SteeringAngleinput1_Ad/1
  SAS_SteeringAngleinput1_C/1 -> SAS_SteeringAngleinput1_P/2
  Demux/1 -> SAS_SteeringAngleinput1_P/1
  SAS_SteeringAngle_sat/1 -> SAS_SteeringAngle_Out/1
  SAS_SteeringAngle_Ad/1 -> SAS_SteeringAngle_sat/1
  SAS_SteeringAngle_O/1 -> SAS_SteeringAngle_Ad/2
  SAS_SteeringAngle_F/1 -> SAS_SteeringAngle_Ad/1

== system VCU_CS75_9_30/长安CS75底盘程序，20ms一次/BSW_Input/DBC转化的messages（存底）/ReceiveMessages14/SCM_3B8 ==
  input : Inport
  Demux : Demux  Outputs=8
  SCM_ACCCancel_Ad : Sum
  SCM_ACCCancel_Convert : DataTypeConversion  OutDataTypeStr=uint32
  SCM_ACCCancel_F : Gain
  SCM_ACCCancel_L : simulink/Logic and Bit Operations/Bitwise Operator  logicop=AND  UseBitMask=on  BitMask=4  BitMaskRealWorld=Stored Integer
  SCM_ACCCancel_O : Constant  Value=0  OutDataTypeStr=single
  SCM_ACCCancel_S : ArithShift  BitShiftNumber=2
  SCM_ACCCancel_Sub : Subsystem
  SCM_ACCCancel_sat : Saturate  UpperLimit=0  LowerLimit=0
  SCM_ACCCancelcv : DataTypeConversion
  SCM_ACCOn_Ad : Sum
  SCM_ACCOn_Convert : DataTypeConversion  OutDataTypeStr=uint32
  SCM_ACCOn_F : Gain
  SCM_ACCOn_L : simulink/Logic and Bit Operations/Bitwise Operator  logicop=AND  UseBitMask=on  BitMask=1  BitMaskRealWorld=Stored Integer
  SCM_ACCOn_O : Constant  Value=0  OutDataTypeStr=single
  SCM_ACCOn_S : ArithShift
  SCM_ACCOn_Sub : Subsystem
  SCM_ACCOn_sat : Saturate  UpperLimit=0  LowerLimit=0
  SCM_ACCOncv : DataTypeConversion
  SCM_IACCOn_Ad : Sum
  SCM_IACCOn_Convert : DataTypeConversion  OutDataTypeStr=uint32
  SCM_IACCOn_F : Gain
  SCM_IACCOn_L : simulink/Logic and Bit Operations/Bitwise Operator  logicop=AND  UseBitMask=on  BitMask=16  BitMaskRealWorld=Stored Integer
  SCM_IACCOn_O : Constant  Value=0  OutDataTypeStr=single
  SCM_IACCOn_S : ArithShift  BitShiftNumber=4
  SCM_IACCOn_Sub : Subsystem
  SCM_IACCOn_sat : Saturate  UpperLimit=0  LowerLimit=0
  SCM_IACCOncv : DataTypeConversion
  SCM_Resume_Ad : Sum
  SCM_Resume_Convert : DataTypeConversion  OutDataTypeStr=uint32
  SCM_Resume_F : Gain
  SCM_Resume_L : simulink/Logic and Bit Operations/Bitwise Operator  logicop=AND  UseBitMask=on  BitMask=16  BitMaskRealWorld=Stored Integer
  SCM_Resume_O : Constant  Value=0  OutDataTypeStr=single
  SCM_Resume_S : ArithShift  BitShiftNumber=4
  SCM_Resume_Sub : Subsystem
  SCM_Resume_sat : Saturate  UpperLimit=0  LowerLimit=0
  SCM_Resumecv : DataTypeConversion
  SCM_Speeddecrease_Ad : Sum
  SCM_Speeddecrease_Convert : DataTypeConversion  OutDataTypeStr=uint32
  SCM_Speeddecrease_F : Gain
  SCM_Speeddecrease_L : simulink/Logic and Bit Operations/Bitwise Operator  logicop=AND  UseBitMask=on  BitMask=64  BitMaskRealWorld=Stored Integer
  SCM_Speeddecrease_O : Constant  Value=0  OutDataTypeStr=single
  SCM_Speeddecrease_S : ArithShift  BitShiftNumber=6
  SCM_Speeddecrease_Sub : Subsystem
  SCM_Speeddecrease_sat : Saturate  UpperLimit=0  LowerLimit=0
  SCM_Speeddecreasecv : DataTypeConversion
  SCM_TimeGap_Ad : Sum
  SCM_TimeGap_Convert : DataTypeConversion  OutDataTypeStr=uint32
  SCM_TimeGap_F : Gain
  SCM_TimeGap_L : simulink/Logic and Bit Operations/Bitwise Operator  logicop=AND  UseBitMask=on  BitMask=1  BitMaskRealWorld=Stored Integer
  SCM_TimeGap_O : Constant  Value=0  OutDataTypeStr=single
  SCM_TimeGap_S : ArithShift
  SCM_TimeGap_Sub : Subsystem
  SCM_TimeGap_sat : Saturate  UpperLimit=0  LowerLimit=0
  SCM_TimeGapcv : DataTypeConversion
  SCM_ACCOn_Out : Outport
  SCM_ACCCancel_Out : Outport  Port=2
  SCM_Resume_Out : Outport  Port=3
  SCM_Speeddecrease_Out : Outport  Port=4
  SCM_TimeGap_Out : Outport  Port=5
  SCM_IACCOn_Out : Outport  Port=6
  wires:
  input/1 -> Demux/1
  SCM_IACCOncv/1 -> SCM_IACCOn_F/1
  SCM_IACCOn_S/1 -> SCM_IACCOncv/1
  SCM_IACCOn_L/1 -> SCM_IACCOn_S/1
  SCM_IACCOn_Convert/1 -> SCM_IACCOn_L/1
  SCM_IACCOn_Sub/1(Out1) -> SCM_IACCOn_Convert/1
  SCM_IACCOn_sat/1 -> SCM_IACCOn_Out/1
  SCM_IACCOn_Ad/1 -> SCM_IACCOn_sat/1
  SCM_IACCOn_O/1 -> SCM_IACCOn_Ad/2
  SCM_IACCOn_F/1 -> SCM_IACCOn_Ad/1
  SCM_TimeGapcv/1 -> SCM_TimeGap_F/1
  SCM_TimeGap_S/1 -> SCM_TimeGapcv/1
  SCM_TimeGap_L/1 -> SCM_TimeGap_S/1
  SCM_TimeGap_Convert/1 -> SCM_TimeGap_L/1
  SCM_TimeGap_Sub/1(Out1) -> SCM_TimeGap_Convert/1
  Demux/2 -> SCM_IACCOn_Sub/1(In1), SCM_TimeGap_Sub/1(In1)
  SCM_TimeGap_sat/1 -> SCM_TimeGap_Out/1
  SCM_TimeGap_Ad/1 -> SCM_TimeGap_sat/1
  SCM_TimeGap_O/1 -> SCM_TimeGap_Ad/2
  SCM_TimeGap_F/1 -> SCM_TimeGap_Ad/1
  SCM_Speeddecreasecv/1 -> SCM_Speeddecrease_F/1
  SCM_Speeddecrease_S/1 -> SCM_Speeddecreasecv/1
  SCM_Speeddecrease_L/1 -> SCM_Speeddecrease_S/1
  SCM_Speeddecrease_Convert/1 -> SCM_Speeddecrease_L/1
  SCM_Speeddecrease_Sub/1(Out1) -> SCM_Speeddecrease_Convert/1
  SCM_Speeddecrease_sat/1 -> SCM_Speeddecrease_Out/1
  SCM_Speeddecrease_Ad/1 -> SCM_Speeddecrease_sat/1
  SCM_Speeddecrease_O/1 -> SCM_Speeddecrease_Ad/2
  SCM_Speeddecrease_F/1 -> SCM_Speeddecrease_Ad/1
  SCM_Resumecv/1 -> SCM_Resume_F/1
  SCM_Resume_S/1 -> SCM_Resumecv/1
  SCM_Resume_L/1 -> SCM_Resume_S/1
  SCM_Resume_Convert/1 -> SCM_Resume_L/1
  SCM_Resume_Sub/1(Out1) -> SCM_Resume_Convert/1
  SCM_Resume_sat/1 -> SCM_Resume_Out/1
  SCM_Resume_Ad/1 -> SCM_Resume_sat/1
  SCM_Resume_O/1 -> SCM_Resume_Ad/2
  SCM_Resume_F/1 -> SCM_Resume_Ad/1
  SCM_ACCCancelcv/1 -> SCM_ACCCancel_F/1
  SCM_ACCCancel_S/1 -> SCM_ACCCancelcv/1
  SCM_ACCCancel_L/1 -> SCM_ACCCancel_S/1
  SCM_ACCCancel_Convert/1 -> SCM_ACCCancel_L/1
  SCM_ACCCancel_Sub/1(Out1) -> SCM_ACCCancel_Convert/1
  SCM_ACCCancel_sat/1 -> SCM_ACCCancel_Out/1
  SCM_ACCCancel_Ad/1 -> SCM_ACCCancel_sat/1
  SCM_ACCCancel_O/1 -> SCM_ACCCancel_Ad/2
  SCM_ACCCancel_F/1 -> SCM_ACCCancel_Ad/1
  SCM_ACCOncv/1 -> SCM_ACCOn_F/1
  SCM_ACCOn_S/1 -> SCM_ACCOncv/1
  SCM_ACCOn_L/1 -> SCM_ACCOn_S/1
  SCM_ACCOn_Convert/1 -> SCM_ACCOn_L/1
  SCM_ACCOn_Sub/1(Out1) -> SCM_ACCOn_Convert/1
  Demux/1 -> SCM_Speeddecrease_Sub/1(In1), SCM_Resume_Sub/1(In1), SCM_ACCCancel_Sub/1(In1), SCM_ACCOn_Sub/1(In1)
  SCM_ACCOn_sat/1 -> SCM_ACCOn_Out/1
  SCM_ACCOn_Ad/1 -> SCM_ACCOn_sat/1
  SCM_ACCOn_O/1 -> SCM_ACCOn_Ad/2
  SCM_ACCOn_F/1 -> SCM_ACCOn_Ad/1

== system VCU_CS75_9_30/长安CS75底盘程序，20ms一次/BSW_Input/DBC转化的messages（存底）/ReceiveMessages15/SRS_005 ==
  input : Inport
  Demux : Demux  Outputs=8
  SRS_DriverBuckleSwitchStatus_Ad : Sum
  SRS_DriverBuckleSwitchStatus_Convert : DataTypeConversion  OutDataTypeStr=uint32
  SRS_DriverBuckleSwitchStatus_F : Gain
  SRS_DriverBuckleSwitchStatus_L : simulink/Logic and Bit Operations/Bitwise Operator  logicop=AND  UseBitMask=on  BitMask=192  BitMaskRealWorld=Stored Integer
  SRS_DriverBuckleSwitchStatus_O : Constant  Value=0  OutDataTypeStr=single
  SRS_DriverBuckleSwitchStatus_S : ArithShift  BitShiftNumber=6
  SRS_DriverBuckleSwitchStatus_Sub : Subsystem
  SRS_DriverBuckleSwitchStatus_sat : Saturate  UpperLimit=3  LowerLimit=0
  SRS_DriverBuckleSwitchStatuscv : DataTypeConversion
  SRS_RollingCounter_Ad : Sum
  SRS_RollingCounter_Convert : DataTypeConversion  OutDataTypeStr=uint32
  SRS_RollingCounter_F : Gain
  SRS_RollingCounter_L : simulink/Logic and Bit Operations/Bitwise Operator  logicop=AND  UseBitMask=on  BitMask=15  BitMaskRealWorld=Stored Integer
  SRS_RollingCounter_O : Constant  Value=0  OutDataTypeStr=single
  SRS_RollingCounter_S : ArithShift
  SRS_RollingCounter_Sub : Subsystem
  SRS_RollingCounter_sat : Saturate  UpperLimit=15  LowerLimit=0
  SRS_RollingCountercv : DataTypeConversion
  SRS_DriverBuckleSwitchStatus_Out : Outport
  SRS_RollingCounter_Out : Outport  Port=2
  wires:
  input/1 -> Demux/1
  SRS_RollingCountercv/1 -> SRS_RollingCounter_F/1
  SRS_RollingCounter_S/1 -> SRS_RollingCountercv/1
  SRS_RollingCounter_L/1 -> SRS_RollingCounter_S/1
  SRS_RollingCounter_Convert/1 -> SRS_RollingCounter_L/1
  SRS_RollingCounter_Sub/1(Out1) -> SRS_RollingCounter_Convert/1
  Demux/4 -> SRS_RollingCounter_Sub/1(In1)
  SRS_RollingCounter_sat/1 -> SRS_RollingCounter_Out/1
  SRS_RollingCounter_Ad/1 -> SRS_RollingCounter_sat/1
  SRS_RollingCounter_O/1 -> SRS_RollingCounter_Ad/2
  SRS_RollingCounter_F/1 -> SRS_RollingCounter_Ad/1
  SRS_DriverBuckleSwitchStatuscv/1 -> SRS_DriverBuckleSwitchStatus_F/1
  SRS_DriverBuckleSwitchStatus_S/1 -> SRS_DriverBuckleSwitchStatuscv/1
  SRS_DriverBuckleSwitchStatus_L/1 -> SRS_DriverBuckleSwitchStatus_S/1
  SRS_DriverBuckleSwitchStatus_Convert/1 -> SRS_DriverBuckleSwitchStatus_L/1
  SRS_DriverBuckleSwitchStatus_Sub/1(Out1) -> SRS_DriverBuckleSwitchStatus_Convert/1
  Demux/2 -> SRS_DriverBuckleSwitchStatus_Sub/1(In1)
  SRS_DriverBuckleSwitchStatus_sat/1 -> SRS_DriverBuckleSwitchStatus_Out/1
  SRS_DriverBuckleSwitchStatus_Ad/1 -> SRS_DriverBuckleSwitchStatus_sat/1
  SRS_DriverBuckleSwitchStatus_O/1 -> SRS_DriverBuckleSwitchStatus_Ad/2
  SRS_DriverBuckleSwitchStatus_F/1 -> SRS_DriverBuckleSwitchStatus_Ad/1
